simulink model "ElectricPowertrain"  (R2023b)
settings: Solver=FixedStepDiscrete  StartTime=0.0  StopTime=Inf  FixedStep=1e-3  RelTol=1e-3
undefined symbols (not defined in the file): BServiceDisconnectNeg, BServiceDisconnectPos, tSim
settings Model: DataDictionary=ElectricPowertrain_data.sldd  PacingRate=1000  Creator=Elio  LastModifiedBy=Elio
settings SFSimCC: SimTargetLang=C++

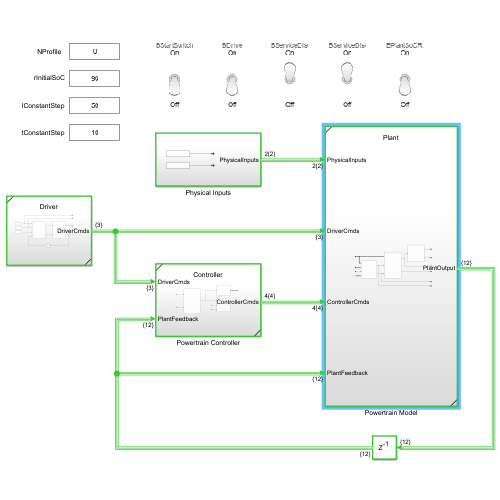
[thumbnail: Simulink's stored preview of the top-level diagram]
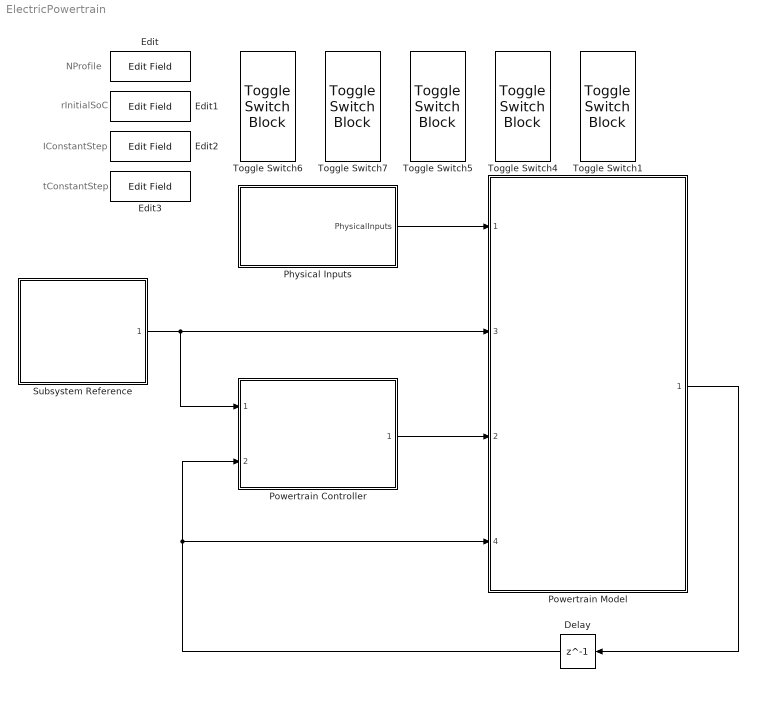
== system ElectricPowertrain ==
  note: NProfile
  note: rInitialSoC
  note: IConstantStep
  note: tConstantStep
  Delay : Delay  DelayLength=1
  Edit{,1..3} (4 alike) : EditField  LabelPosition=Hide  ShowInitialText=on  Alignment=Center
  Physical Inputs : Subsystem
  Powertrain Controller : Subsystem  ReferencedSubsystem=Controller
      settings: PermitHierarchicalResolution=None
  Powertrain Model : Subsystem  ReferencedSubsystem=Plant
      settings: PermitHierarchicalResolution=None  PortSchema="{\"entries\":[{\"content\":{\"sides\":[{\"content\":{\"connectorIds\":[\"In1\",\"In3\",\"In2\",\"In4\"]},\"type\":\"ConnectorPlacement.EquallySpacedRectSide\",\"uuid\":\"7f0793ce-a99d-424a-b534-09cc8e7f96d6\"},{\"content\":{\"connectorIds\":[\"Out1\"],\"side\":\"RIGHT\"},\"type\":\"ConnectorPlacement.EquallySpacedRectSide\",\"uuid\":\"9744bc4c-d77e-4732-9b80-6b439d1824ed\"},{\"content\":{\"side\":\"TOP\"},\"type\":\"ConnectorPlacement.EquallySpacedRectSide\",\"uuid\":\"1db6836e-5eea-4951-9b9a-f244a01439b8\"}]},\"type\":\"ConnectorPlacement.EquallySpacedConnector\",\"uuid\":\"a69c2ff2-1f1a-4e2a-a6fe-777bc8fa3086\"}],\"packageUris\":[\"http://schema.mathworks.com/mf0/Connector/R2020b\"],\"version\":\"1.0\"}"
  Subsystem Reference : Subsystem  ReferencedSubsystem=Driver
  Toggle Switch{1,4..7} (5 alike) : ToggleSwitchBlock
      settings: Values={{'Off', 'On'}, [0 1]}
  wires:
  Powertrain Model/1 -> Delay/1
  Delay/1 -> Powertrain Model/4, Powertrain Controller/2
  Physical Inputs/1(PhysicalInputs) -> Powertrain Model/1
  Subsystem Reference/1 -> Powertrain Controller/1, Powertrain Model/3
  Powertrain Controller/1 -> Powertrain Model/2

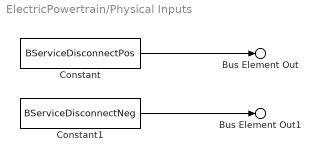
== system ElectricPowertrain/Physical Inputs ==
  Constant : Constant  Value=BServiceDisconnectPos  SampleTime=tSim
  Constant1 : Constant  Value=BServiceDisconnectNeg  SampleTime=tSim
  Bus Element Out : Outport  PortName=PhysicalInputs  Element=BServiceDisconnectPos
  Bus Element Out1 : Outport  PortName=PhysicalInputs  Element=BServiceDisconnectNeg
  wires:
  Constant/1 -> Bus Element Out/1
  Constant1/1 -> Bus Element Out1/1
